simulink model "SYSTEMS"  (R2024b)
settings: Solver=FixedStepDiscrete  StartTime=0.0  StopTime=1  FixedStep=0.001  RelTol=1e-3  EnableMultiTasking=on
settings Model: DataDictionary=Master_Dictionary.sldd  EnableAccessToBaseWorkspace=off  Creator=torni  LastModifiedBy=oxbro
settings SolverCC: AlgebraicLoopSolver=TrustRegion
settings DataIOCC: ReturnWorkspaceOutputs=off
settings OptimizationCC: DefaultParameterBehavior=Inlined  EnhancedBackFolding=on  PassReuseOutputArgsAs=Individual arguments  ZeroExternalMemoryAtStartup=off  ZeroInternalMemoryAtStartup=off  MaxStackSize=512  OptimizeBlockOrder=speed  DifferentSizesBufferReuse=on  OptimizationCustomize=off  EfficientTunableParamExpr=on
settings DebuggingCC: ParameterTunabilityLossMsg=error  UnconnectedInputMsg=warning  UnconnectedOutputMsg=warning  UnconnectedLineMsg=warning  ArithmeticOperatorsInVariantConditions=warning
settings HardwareCC: ProdBitPerPointer=32  ProdBitPerSizeT=32  ProdBitPerPtrDiffT=32  ProdLargestAtomicInteger=Long  ProdLargestAtomicFloat=Double  ProdWordSize=32  ProdLongLongMode=on  ProdHWDeviceType=ARM Compatible->ARM Cortex-M
settings ModelReferenceCC: EnableRefExpFcnMdlSchedulingChecks=on
settings SFSimCC: MATLABDynamicMemAlloc=off  CustomCodeUndefinedFunction=UseInterfaceOnly
settings RTWCC: Description=Embedded Coder  SystemTargetFile=ert.tlc  HardwareBoard=STM32H7xx Based (Single-core)  TemplateMakefile=ert_default_tmf  CustomHeaderCode="#include \"stm32h7xx_ll_tim.h\""  CustomInitializer=LL_TIM_EnableCounter(TIM2);  Toolchain=GNU Tools for ARM Embedded Processors  GPUComputeCapability=3.5
settings CodeAppCC: ForceParamTrailComments=on  IgnoreCustomStorageClasses=off  OperatorAnnotations=on  SimulinkDataObjDesc=on  SFDataObjDesc=on  InsertBlockDesc=on
settings ERTTargetCC: TargetLangStandard=C99 (ISO)  CodeReplacementLibrary=ARM Cortex-M  ExtModeTransport=3  ExtModeStaticAlloc=on  ExtModeStaticAllocSize=2048  ExtModeMexFile=ext_xcp  ExtModeIntrfLevel=Level2 - Open

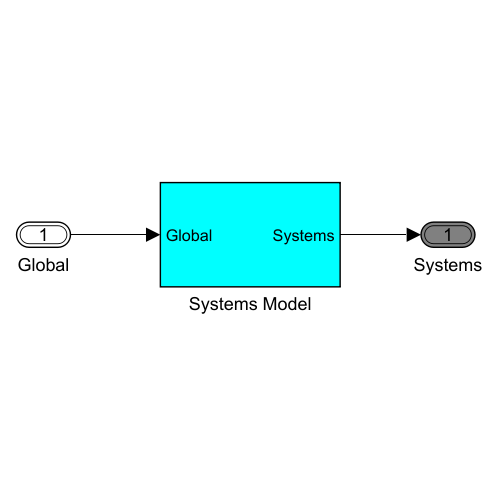
[thumbnail: Simulink's stored preview of the top-level diagram]
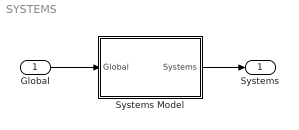
== system SYSTEMS ==
  "Global " : Inport  OutDataTypeStr=Bus: Global  Interpolate=off
  Systems Model : Subsystem
  Systems : Outport  OutDataTypeStr=Bus: Systems  VectorParamsAs1DForOutWhenUnconnected=off
  wires:
  "Global "/1 -> Systems Model/1(Global)
  Systems Model/1(Systems) -> Systems/1

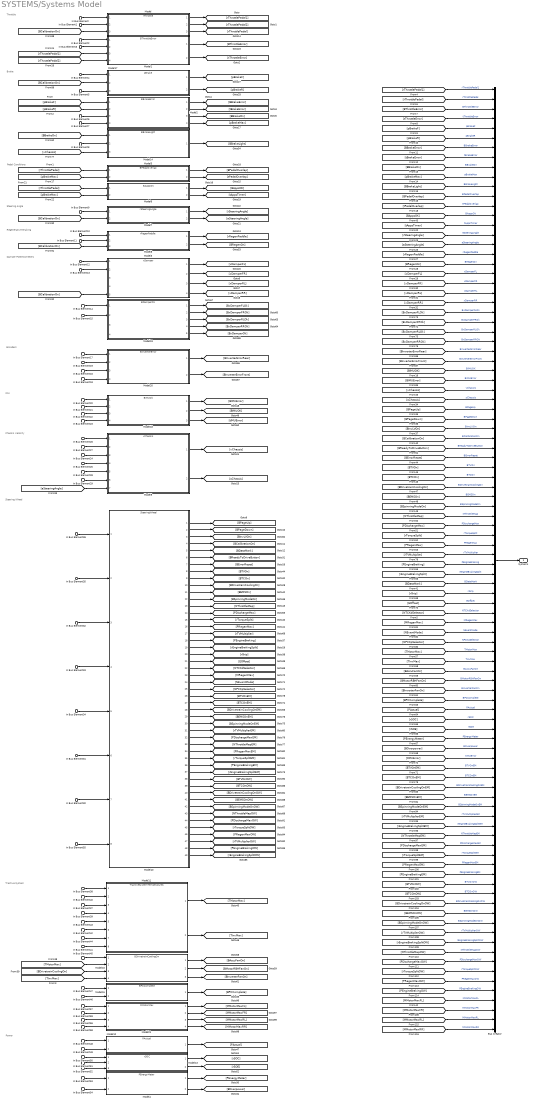
== system SYSTEMS/Systems Model ==
  note: Power
  note: Pedal Conditions
  note: IMU
  note: Damper Potentiometers
  note: Regenerative Braking
  note: Steering Wheel
  note: Steering Angle
  note: Brake
  note: Throttle
  note: Tractive System
  note: Chassis Velocity
  note: Encoders
  In Bus Element : Inport  PortName=Global  Element=SensorSignals.VThrottlePedal1
  In Bus Element2 : Inport  PortName=Global  Element=SensorSignals.VThrottlePedal1
  In Bus Element1 : Inport  PortName=Global  Element=SensorSignals.VThrottlePedal2
  In Bus Element3 : Inport  PortName=Global  Element=SensorSignals.VThrottlePedal2
  In Bus Element4 : Inport  PortName=Global  Element=SensorSignals.VBrakeF
  In Bus Element6 : Inport  PortName=Global  Element=SensorSignals.VBrakeF
  In Bus Element5 : Inport  PortName=Global  Element=SensorSignals.VBrakeR
  In Bus Element7 : Inport  PortName=Global  Element=SensorSignals.VBrakeR
  In Bus Element9 : Inport  PortName=Global  Element=SensorSignals.VSteeringAngle
  In Bus Element10 : Inport  PortName=Global  Element=SensorSignals.VRegenPaddle1
  In Bus Element11 : Inport  PortName=Global  Element=SensorSignals.VRegenPaddle2
  In Bus Element12 : Inport  PortName=Global  Element=SensorSignals.VDamperPotentiometerFL
  In Bus Element14 : Inport  PortName=Global  Element=SensorSignals.VDamperPotentiometerFL
  In Bus Element13 : Inport  PortName=Global  Element=SensorSignals.VDamperPotentiometerFR
  In Bus Element15 : Inport  PortName=Global  Element=SensorSignals.VDamperPotentiometerFR
  In Bus Element30 : Inport  PortName=Global  Element=SensorSignals.BSteeringWheelButton1
  In Bus Element31 : Inport  PortName=Global  Element=SensorSignals.BSteeringWheelButton2
  In Bus Element32 : Inport  PortName=Global  Element=SensorSignals.BSteeringWheelButton3
  In Bus Element33 : Inport  PortName=Global  Element=SensorSignals.BSteeringWheelButton4
  In Bus Element34 : Inport  PortName=Global  Element=SensorSignals.NPageSelectRotary
  In Bus Element35 : Inport  PortName=Global  Element=SensorSignals.NParameterRotary
  In Bus Element36 : Inport  PortName=Global  Element=SensorSignals.NEventModeRotary
  In Bus Element8 : Inport  PortName=Global  Element=GPSIMUSignals.gLongitudinalIMU
  In Bus Element20 : Inport  PortName=Global  Element=GPSIMUSignals.gLongitudinalIMU
  In Bus Element29 : Inport  PortName=Global  Element=GPSIMUSignals.gLongitudinalIMU
  In Bus Element21 : Inport  PortName=Global  Element=GPSIMUSignals.gLateralIMU
  In Bus Element28 : Inport  PortName=Global  Element=GPSIMUSignals.gLateralIMU
  In Bus Element22 : Inport  PortName=Global  Element=GPSIMUSignals.nYawRateIMU
  In Bus Element23 : Inport  PortName=Global  Element=GPSIMUSignals.gVerticalIMU
  In Bus Element16 : Inport  PortName=Global  Element=InverterSignals.InverterRLSignals.NInvDTCRL
  In Bus Element37 : Inport  PortName=Global  Element=InverterSignals.InverterRLSignals.TMotorRL
  In Bus Element44 : Inport  PortName=Global  Element=InverterSignals.InverterRLSignals.TInvRL
  In Bus Element47 : Inport  PortName=Global  Element=InverterSignals.InverterRLSignals.VDCInvRL
  In Bus Element48 : Inport  PortName=Global  Element=InverterSignals.InverterRLSignals.VDCInvRL
  In Bus Element56 : Inport  PortName=Global  Element=InverterSignals.InverterRLSignals.nMotorRL
  In Bus Element17 : Inport  PortName=Global  Element=InverterSignals.InverterFLSignals.NInvDTCFL
  In Bus Element38 : Inport  PortName=Global  Element=InverterSignals.InverterFLSignals.TMotorFL
  In Bus Element43 : Inport  PortName=Global  Element=InverterSignals.InverterFLSignals.TInvFL
  In Bus Element57 : Inport  PortName=Global  Element=InverterSignals.InverterFLSignals.nMotorFL
  In Bus Element18 : Inport  PortName=Global  Element=InverterSignals.InverterRRSignals.NInvDTCRR
  In Bus Element39 : Inport  PortName=Global  Element=InverterSignals.InverterRRSignals.TMotorRR
  In Bus Element41 : Inport  PortName=Global  Element=InverterSignals.InverterRRSignals.TInvRR
  In Bus Element58 : Inport  PortName=Global  Element=InverterSignals.InverterRRSignals.nMotorRR
  In Bus Element19 : Inport  PortName=Global  Element=InverterSignals.InverterFRSignals.NInvDTCFR
  In Bus Element40 : Inport  PortName=Global  Element=InverterSignals.InverterFRSignals.TMotorFR
  In Bus Element42 : Inport  PortName=Global  Element=InverterSignals.InverterFRSignals.TInvFR
  In Bus Element59 : Inport  PortName=Global  Element=InverterSignals.InverterFRSignals.nMotorFR
  In Bus Element24 : Inport  PortName=Global  Element=WheelSpeeds.vWheelRL
  In Bus Element25 : Inport  PortName=Global  Element=WheelSpeeds.vWheelRR
  In Bus Element26 : Inport  PortName=Global  Element=WheelSpeeds.vWheelFL
  In Bus Element27 : Inport  PortName=Global  Element=WheelSpeeds.vWheelFR
  In Bus Element45 : Inport  PortName=Global  Element=BMSSignals.TCellMax
  In Bus Element46 : Inport  PortName=Global  Element=BMSSignals.VDCAccumulator
  In Bus Element51 : Inport  PortName=Global  Element=BMSSignals.VDCAccumulator
  In Bus Element53 : Inport  PortName=Global  Element=BMSSignals.VDCAccumulator
  In Bus Element49 : Inport  PortName=Global  Element=BMSSignals.IIVTS
  In Bus Element50 : Inport  PortName=Global  Element=BMSSignals.IIVTS
  In Bus Element54 : Inport  PortName=Global  Element=BMSSignals.IIVTS
  In Bus Element52 : Inport  PortName=Global  Element=BMSSignals.VCellMin
  In Bus Element55 : Inport  PortName=Global  Element=Stateflow.NCarState
  Bus Creator : BusCreator  Inputs=98  OutDataTypeStr=Bus: Systems
  Model : ModelReference  ModelNameDialog=rThrottle  SimulationMode=Normal  ModelReferenceVersion=13.0
  Model1 : ModelReference  ModelNameDialog=BThrottleError  SimulationMode=Normal  ModelReferenceVersion=13.0
  Model10 : ModelReference  ModelNameDialog=SteeringWheel.slx  SimulationMode=Normal  ModelReferenceVersion=13.0
  Model11 : ModelReference  ModelNameDialog=TractiveSystemTemperatures.slx  SimulationMode=Normal  ModelReferenceVersion=13.0
  Model12 : ModelReference  ModelNameDialog=PActual.slx  SimulationMode=Normal  ModelReferenceVersion=13.0
  Model13 : ModelReference  ModelNameDialog=rSOC.slx  SimulationMode=Normal  ModelReferenceVersion=13.0
  Model14 : ModelReference  ModelNameDialog=BBrakeLight.slx  SimulationMode=Normal  ModelReferenceVersion=13.0
  Model15 : ModelReference  ModelNameDialog=BPCComplete  SimulationMode=Normal  ModelReferenceVersion=13.0
  Model16 : ModelReference  ModelNameDialog=BDrivetrainCoolingOn.slx  SimulationMode=Normal  ModelReferenceVersion=13.0
  Model17 : ModelReference  ModelNameDialog=pBrake  SimulationMode=Normal  ModelReferenceVersion=13.0
  Model18 : ModelReference  ModelNameDialog=BIMUOk  SimulationMode=Normal  ModelReferenceVersion=13.0
  Model19 : ModelReference  ModelNameDialog=BDamperOk.slx  SimulationMode=Normal  ModelReferenceVersion=13.0
  Model2 : ModelReference  ModelNameDialog=BBrakeError  SimulationMode=Normal  ModelReferenceVersion=13.0
  Model20 : ModelReference  ModelNameDialog=BInverterError.slx  SimulationMode=Normal  ModelReferenceVersion=13.0
  Model21 : ModelReference  ModelNameDialog=MMotorMax.slx  SimulationMode=Normal  ModelReferenceVersion=13.0
  Model3 : ModelReference  ModelNameDialog=xDamper  SimulationMode=Normal  ModelReferenceVersion=13.0
  Model4 : ModelReference  ModelNameDialog=PEnergyMeter  SimulationMode=Normal  ModelReferenceVersion=13.2
  Model5 : ModelReference  ModelNameDialog=BPedalOverlap  SimulationMode=Normal  ModelReferenceVersion=13.0
  Model6 : ModelReference  ModelNameDialog=BAppsOK.slx  SimulationMode=Normal  ModelReferenceVersion=13.0
  Model7 : ModelReference  ModelNameDialog=rSteeringAngle.slx  SimulationMode=Normal  ModelReferenceVersion=13.0
  Model8 : ModelReference  ModelNameDialog=rRegenPaddle.slx  SimulationMode=Normal  ModelReferenceVersion=13.0
  Model9 : ModelReference  ModelNameDialog=vChassis.slx  SimulationMode=Normal  ModelReferenceVersion=13.0
  Systems : Outport  OutDataTypeStr=Bus: Systems  VectorParamsAs1DForOutWhenUnconnected=off  LockScale=on
  wires:
  In Bus Element/1 -> Model/1
  In Bus Element1/1 -> Model/2
  In Bus Element3/1 -> Model1/2
  In Bus Element2/1 -> Model1/1
  Model/1 -> [rThrottlePedal1]
  Model/2 -> [rThrottlePedal2]
  [rThrottlePedal1] -> Model1/3
  [rThrottlePedal2] -> Model1/4
  Model1/1 -> [BThrottleError]
  Model2/1 -> [BBrakeError]
  ? -> Model3/4
  ? -> Model3/3
  In Bus Element13/1 -> Model3/2
  In Bus Element12/1 -> Model3/1
  Model1/2 -> [tThrottleError]
  Model2/2 -> [tBrakeError]
  Model3/1 -> [xDamperFL]
  Model3/2 -> [xDamperFR]
  Model3/4 -> [xDamperRR]
  Model3/3 -> [xDamperRL]
  [rThrottlePedal] -> Model5/1
  Model5/2 -> [tPedalOverlap]
  Model5/1 -> [BPedalOverlap]
  Bus Creator/1 -> Systems/1
  Model2/3 -> [BBrakeOn]
  Model2/4 -> [pBrakeMax]
  [pBrakeMax] -> Model6/2
  [pBrakeMax] -> Model5/2
  Model6/1 -> [BAppsOK]
  Model6/2 -> [tAppsTimer]
  [rThrottlePedal] -> Model6/1
  Model/3 -> [rThrottlePedal]
  Model8/1 -> [rRegenPaddle]
  Model7/1 -> [rSteeringAngle]
  Model7/2 -> [aSteeringAngle]
  Model9/2 -> [sChassis]
  In Bus Element9/1 -> Model7/1
  Model9/1 -> [vChassis]
  Model12/1 -> [PActual]
  Model13/1 -> [rSOC]
  Model13/2 -> [rSOE]
  Model8/2 -> [BRegenOn]
  [BBrakeOn] -> Model14/1
  Model14/1 -> [BBrakeLight]
  Model16/1 -> [BAccuFanOn]
  Model16/2 -> [BMotorRBHFanOn]
  Model16/3 -> [BInverterFanOn]
  In Bus Element8/1 -> Model14/2
  [vChassis] -> Model14/3
  Model11/2 -> [TInvMax]
  Model11/1 -> [TMotorMax]
  Model17/1 -> [pBrakeF]
  Model17/2 -> [pBrakeR]
  [pBrakeR] -> Model2/2
  [pBrakeF] -> Model2/1
  [TInvMax] -> Model16/4
  [TMotorMax] -> Model16/2
  [BDrivetrainCoolingOn] -> Model16/3
  Model4/1 -> [PEnergyMeter]
  Model4/2 -> [BOverpower]
  Model15/1 -> [BPCComplete]
  [rThrottlePedal1] -> Bus Creator/1  "rThrottlePedal1"
  [BCalibrationOn] -> Model/3
  [BCalibrationOn] -> Model17/2
  [BCalibrationOn] -> Model7/2
  [BCalibrationOn] -> Model8/3
  In Bus Element11/1 -> Model8/2
  In Bus Element10/1 -> Model8/1
  [BCalibrationOn] -> Model3/5
  In Bus Element29/1 -> Model9/6
  In Bus Element28/1 -> Model9/5
  In Bus Element27/1 -> Model9/2
  In Bus Element24/1 -> Model9/3
  In Bus Element26/1 -> Model9/1
  In Bus Element25/1 -> Model9/4
  In Bus Element20/1 -> Model18/1
  In Bus Element21/1 -> Model18/2
  In Bus Element22/1 -> Model18/3
  Model18/1 -> [BIMUError]
  In Bus Element4/1 -> Model17/1
  In Bus Element5/1 -> Model17/3
  In Bus Element6/1 -> Model2/3
  In Bus Element7/1 -> Model2/4
  Model18/2 -> [BIMUOK]
  Model18/3 -> [tIMUError]
  [aSteeringAngle] -> Model9/7
  In Bus Element15/1 -> Model19/2
  ? -> Model19/4
  ? -> Model19/3
  In Bus Element14/1 -> Model19/1
  Model19/1 -> [BxDamperFLOk]
  Model19/2 -> [BxDamperFROk]
  Model19/4 -> [BxDamperRROk]
  Model19/3 -> [BxDamperRLOk]
  Model19/5 -> [BxDamperOk]
  In Bus Element19/1 -> Model20/2
  In Bus Element16/1 -> Model20/3
  In Bus Element17/1 -> Model20/1
  In Bus Element18/1 -> Model20/4
  Model20/1 -> [BInverterErrorRear]
  Model20/2 -> [BInverterErrorFront]
  In Bus Element23/1 -> Model18/4
  In Bus Element37/1 -> Model11/3
  In Bus Element40/1 -> Model11/2
  In Bus Element39/1 -> Model11/4
  In Bus Element38/1 -> Model11/1
  In Bus Element43/1 -> Model11/5
  In Bus Element41/1 -> Model11/8
  In Bus Element42/1 -> Model11/6
  In Bus Element44/1 -> Model11/7
  In Bus Element47/1 -> Model15/1
  In Bus Element46/1 -> Model15/2
  In Bus Element45/1 -> Model16/1
  In Bus Element48/1 -> Model12/1
  In Bus Element49/1 -> Model12/2
  In Bus Element50/1 -> Model13/1
  In Bus Element51/1 -> Model13/2
  In Bus Element52/1 -> Model13/3
  In Bus Element53/1 -> Model4/1
  In Bus Element54/1 -> Model4/2
  [rThrottlePedal] -> Bus Creator/2  "rThrottlePedal"
  [BThrottleError] -> Bus Creator/3  "BThrottleError"
  [tThrottleError] -> Bus Creator/4  "tThrottleError"
  [pBrakeF] -> Bus Creator/5  "pBrakeF"
  [pBrakeR] -> Bus Creator/6  "pBrakeR"
  [BBrakeError] -> Bus Creator/7  "BBrakeError"
  [tBrakeError] -> Bus Creator/8  "tBrakeError"
  [BBrakeOn] -> Bus Creator/9  "BBrakeOn"
  [pBrakeMax] -> Bus Creator/10  "pBrakeMax"
  [BBrakeLight] -> Bus Creator/11  "BBrakeLight"
  [BPedalOverlap] -> Bus Creator/12  "BPedalOverlap"
  [tPedalOverlap] -> Bus Creator/13  "tPedalOverlap"
  [BAppsOK] -> Bus Creator/14  "BAppsOk"
  [tAppsTimer] -> Bus Creator/15  "tAppsTimer"
  [rSteeringAngle] -> Bus Creator/16  "rSteeringAngle"
  [aSteeringAngle] -> Bus Creator/17  "aSteeringAngle"
  [rRegenPaddle] -> Bus Creator/18  "rRegenPaddle"
  [BRegenOn] -> Bus Creator/19  "BRegenOn"
  [xDamperFL] -> Bus Creator/20  "xDamperFL"
  [xDamperFR] -> Bus Creator/21  "xDamperFR"
  [xDamperRL] -> Bus Creator/22  "xDamperRL"
  [xDamperRR] -> Bus Creator/23  "xDamperRR"
  [BxDamperFLOk] -> Bus Creator/24  "BxDamperFLOk"
  [BxDamperFROk] -> Bus Creator/25  "BxDamperFROk"
  [BxDamperRLOk] -> Bus Creator/26  "BxDamperRLOk"
  [BxDamperRROk] -> Bus Creator/27  "BxDamperRROk"
  [BInverterErrorRear] -> Bus Creator/28  "BInverterErrorRear"
  [BInverterErrorFront] -> Bus Creator/29  "BInverterErrorFront"
  [BIMUOK] -> Bus Creator/30  "BIMUOK"
  [BIMUError] -> Bus Creator/31  "BIMUError"
  [vChassis] -> Bus Creator/32  "vChassis"
  [sChassis] -> Bus Creator/33  "sChassis"
  [BPageUp] -> Bus Creator/34  "BPageUp"
  [BPageDown] -> Bus Creator/35  "BPageDown"
  [BInvLVOn] -> Bus Creator/36  "BInvLVOn"
  [BCalibrationOn] -> Bus Creator/37  "BCalibrationOn"
  [BReadyToDriveButton] -> Bus Creator/38  "BReadyToDriveButton"
  [BErrorReset] -> Bus Creator/39  "BErrorReset"
  [BTVOn] -> Bus Creator/40  "BTVOn"
  [BTCOn] -> Bus Creator/41  "BTCOn"
  [BDrivetrainCoolingOn] -> Bus Creator/42  "BDrivetrainCoolingOn"
  [BEMSOn] -> Bus Creator/43  "BEMSOn"
  [BSpinningModeOn] -> Bus Creator/44  "BSpinningModeOn"
  [NThrottleMap] -> Bus Creator/45  "NThrottleMap"
  [PDischargeMax] -> Bus Creator/46  "PDischargeMax"
  [rTorqueSplit] -> Bus Creator/47  "rTorqueSplit"
  [PRegenMax] -> Bus Creator/48  "PRegenMax"
  [rTVMultiplier] -> Bus Creator/49  "rTVMultiplier"
  [PEngineBraking] -> Bus Creator/50  "PEngineBraking"
  [rEngineBrakingSplit] -> Bus Creator/51  "rEngineBrakingSplit"
  [BDataMark] -> Bus Creator/52  "BDataMark"
  [rGrip] -> Bus Creator/53  "rGrip"
  [EOffset] -> Bus Creator/54  "EOffset"
  [NTCKdSelector] -> Bus Creator/55  "NTCKdSelector"
  [MRegenMax] -> Bus Creator/56  "MRegenMax"
  [NEventMode] -> Bus Creator/57  "NEventMode"
  [NPCKpSelector] -> Bus Creator/58  "NPCKpSelector"
  [TMotorMax] -> Bus Creator/59  "TMotorMax"
  [TInvMax] -> Bus Creator/60  "TInvMax"
  [BAccuFanOn] -> Bus Creator/61  "BAccuFanOn"
  [BInverterFanOn] -> Bus Creator/63  "BInverterFanOn"
  [BPCComplete] -> Bus Creator/64  "BPCComplete"
  [PActual] -> Bus Creator/65  "PActual"
  [rSOC] -> Bus Creator/66  "rSOC"
  [rSOE] -> Bus Creator/67  "rSOE"
  [PEnergyMeter] -> Bus Creator/68  "PEnergyMeter"
  [BOverpower] -> Bus Creator/69  "BOverpower"
  [tIMUError] -> Bus Creator/70  "tIMUError"
  [BTVOnEM] -> Bus Creator/71  "BTVOnEM"
  [BTCOnEM] -> Bus Creator/72  "BTCOnEM"
  [BDrivetrainCoolingOnEM] -> Bus Creator/73  "BDrivetrainCoolingOnEM"
  [BEMSOnEM] -> Bus Creator/74  "BEMSOnEM"
  [BSpinningModeOnEM] -> Bus Creator/75  "BSpinningModeOnEM"
  [rTVMultiplierEM] -> Bus Creator/76  "rTVMultiplierEM"
  [rEngineBrakingSplitEM] -> Bus Creator/77  "rEngineBrakingSplitEM"
  [NThrottleMapEM] -> Bus Creator/78  "NThrottleMapEM"
  [PDischargeMaxEM] -> Bus Creator/79  "PDischargeMaxEM"
  [rTorqueSplitEM] -> Bus Creator/80  "rTorqueSplitEM"
  [PRegenMaxEM] -> Bus Creator/81  "PRegenMaxEM"
  [PEngineBrakingEM] -> Bus Creator/82  "PEngineBrakingEM"
  [BTVOnOW] -> Bus Creator/83  "BTVOnOW"
  [BTCOnOW] -> Bus Creator/84  "BTCOnOW"
  [BEMSOnOW] -> Bus Creator/86  "BEMSOnOW"
  [BDrivetrainCoolingOnOW] -> Bus Creator/85  "BDrivetrainCoolingOnOW"
  [BSpinningModeOnOW] -> Bus Creator/87  "BSpinningModeOnOW"
  [rTVMultiplierOW] -> Bus Creator/88  "rTVMultiplierOW"
  [rEngineBrakingSplitOW] -> Bus Creator/89  "rEngineBrakingSplitOW"
  [NThrottleMapOW] -> Bus Creator/90  "NThrottleMapOW"
  [PDischargeMaxOW] -> Bus Creator/91  "PDischargeMaxOW"
  [rTorqueSplitOW] -> Bus Creator/92  "rTorqueSplitOW"
  [PRegenMaxOW] -> Bus Creator/93  "PRegenMaxOW"
  [PEngineBrakingOW] -> Bus Creator/94  "PEngineBrakingOW"
  In Bus Element36/1 -> Model10/1
  In Bus Element32/1 -> Model10/3
  In Bus Element33/1 -> Model10/4
  In Bus Element34/1 -> Model10/5
  In Bus Element35/1 -> Model10/2
  In Bus Element55/1 -> Model10/8
  In Bus Element31/1 -> Model10/6
  In Bus Element30/1 -> Model10/7
  Model10/1 -> [BPageUp]
  Model10/2 -> [BPageDown]
  Model10/3 -> [BInvLVOn]
  Model10/4 -> [BCalibrationOn]
  Model10/5 -> [BDataMark]
  Model10/6 -> [BReadyToDriveButton]
  Model10/7 -> [BErrorReset]
  Model10/8 -> [BTVOn]
  Model10/9 -> [BTCOn]
  Model10/10 -> [BDrivetrainCoolingOn]
  Model10/11 -> [BEMSOn]
  Model10/12 -> [BSpinningModeOn]
  Model10/13 -> [NThrottleMap]
  Model10/14 -> [PDischargeMax]
  Model10/15 -> [rTorqueSplit]
  Model10/16 -> [PRegenMax]
  Model10/17 -> [rTVMultiplier]
  Model10/18 -> [PEngineBraking]
  Model10/19 -> [rEngineBrakingSplit]
  Model10/20 -> [rGrip]
  Model10/21 -> [EOffset]
  Model10/22 -> [NTCKdSelector]
  Model10/23 -> [MRegenMax]
  Model10/24 -> [NEventMode]
  Model10/25 -> [NPCKpSelector]
  Model10/26 -> [BTVOnEM]
  Model10/27 -> [BTCOnEM]
  Model10/28 -> [BDrivetrainCoolingOnEM]
  Model10/29 -> [BEMSOnEM]
  Model10/30 -> [BSpinningModeOnEM]
  Model10/31 -> [rTVMultiplierEM]
  Model10/33 -> [NThrottleMapEM]
  Model10/35 -> [rTorqueSplitEM]
  Model10/36 -> [PEngineBrakingEM]
  Model10/34 -> [PRegenMaxEM]
  Model10/37 -> [rEngineBrakingSplitEM]
  Model10/32 -> [PDischargeMaxEM]
  Model10/38 -> [BTVOnOW]
  Model10/39 -> [BTCOnOW]
  Model10/40 -> [BDrivetrainCoolingOnOW]
  Model10/41 -> [BEMSOnOW]
  Model10/42 -> [BSpinningModeOnOW]
  Model10/47 -> [rTVMultiplierOW]
  Model10/49 -> [rEngineBrakingSplitOW]
  Model10/48 -> [PEngineBrakingOW]
  Model10/46 -> [PRegenMaxOW]
  Model10/45 -> [rTorqueSplitOW]
  Model10/43 -> [NThrottleMapOW]
  Model10/44 -> [PDischargeMaxOW]
  [BMotorRBHFanOn] -> Bus Creator/62  "BMotorRBHFanOn"
  In Bus Element56/1 -> Model21/3
  In Bus Element57/1 -> Model21/1
  In Bus Element59/1 -> Model21/2
  In Bus Element58/1 -> Model21/4
  Model21/1 -> [MMotorMaxFL]
  Model21/2 -> [MMotorMaxFR]
  Model21/4 -> [MMotorMaxRR]
  Model21/3 -> [MMotorMaxRL]
  [MMotorMaxFL] -> Bus Creator/95  "MMotorMaxFL"
  [MMotorMaxFR] -> Bus Creator/96  "MMotorMaxFR"
  [MMotorMaxRL] -> Bus Creator/97  "MMotorMaxRL"
  [MMotorMaxRR] -> Bus Creator/98  "MMotorMaxRR"
